simulink model "sampleModel2017"  (R2023a)
settings: Solver=VariableStepAuto  StartTime=0.0  StopTime=10.0  RelTol=1e-3
libraries: hdlsllib x4, simulink x3
settings Model: Creator=user1  LastModifiedBy=user1

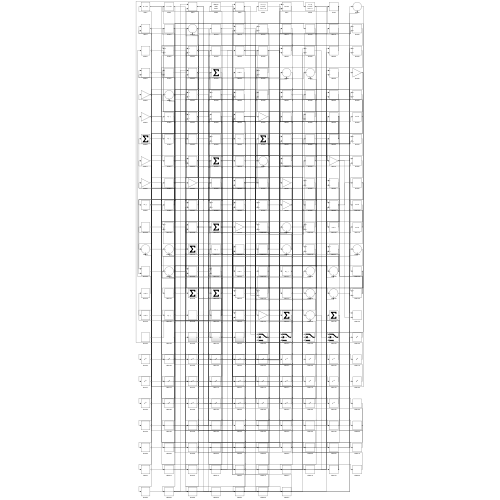
[thumbnail: Simulink's stored preview of the top-level diagram]
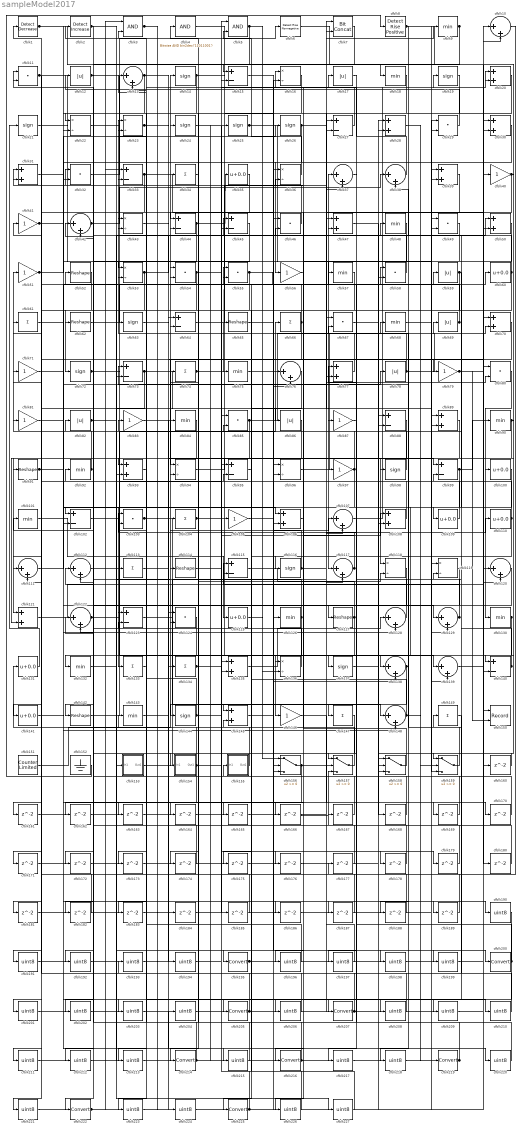
== system sampleModel2017 ==
  cfblk1 : simulink/Logic and Bit Operations/Detect Decrease  vinit=0.0  OutDataTypeStr=boolean
      settings: LibrarySourceBlock=|
      | hdlsllib/Logic and Bit
      | Operations/Detect
      | Decrease
  cfblk{10,13,37..38,42,76,107,111..112,117,120,122,128..129,138..139,148} (17 alike) : Sum  Inputs=|++
  cfblk{35,60,100,109..110,125,131,141} (8 alike) : Bias  Bias=0.0  SaturateOnIntegerOverflow=off
  cfblk{9,18,48,57,68,75,84,90,92,101,126,130,132,143} (14 alike) : MinMax
  cfblk{15,27,33,44..45,64,73,88,95,99,102,115,123,140} (14 alike) : Sum  Inputs=+-
  cfblk{11,29,32,46,49,54..55,58,67,80,85,103,124} (13 alike) : DotProduct  OutDataTypeStr=Inherit: Inherit via internal rule
  cfblk{34,61,66,74,104,113,133..134,147,149} (10 alike) : Sum  Inputs=+
  cfblk{40..41,51,56,71,79,81,83,87,97,105,146} (12 alike) : Gain
  cfblk{20,28,30..31,39,47,50,70,77,89,93,106,108,121,135,145} (16 alike) : Sum
  cfblk{52,62,65,91,114,127,142} (7 alike) : Reshape
  cfblk{14,19,21,24..26,63,72,98,116,137,144} (12 alike) : Signum
  cfblk{16,22..23,36,43,53,94,96,118..119,136} (11 alike) : Product  Inputs=*/  RndMeth=Zero  SaturateOnIntegerOverflow=on
  cfblk{12,17,59,69,78,82,86} (7 alike) : Abs  SaturateOnIntegerOverflow=off
  cfblk150 : Record  FileSettingsInternal="{\"entries\":[{\"content\":{\"excelSettings\":{\"content\":{},\"type\":\"Streamout.ExcelSettings\"}},\"type\":\"Streamout.FileSettingStorage\",\"uuid\":\"\"}],\"packageUris\":[\"http:\\/\\/schema.mathworks.com\\/mf0\\/streamout_blocks\\/R2020a\"],\"version\":\"1.0\"}"  Layout=[1 1]  SignalsInternal="{\"entries\":[{\"content\":{\"signals\":[{\"content\":{\"blockPath\":[],\"dimensions\":[1],\"domain\":\"\",\"lineColor\":\"#a2142f\",\"plots\":[1],\"port\":1,\"signalID\":5993,\"signalName\":\"XY Graph:1\"},\"type\":\"RecordBlkView.Signal\",\"uuid\":\"\"},{\"content\":{\"blockPath\":[],\"dimensions\":[1],\"domain\":\"\",\"lineColor\":\"#139fff\",\"plots\":[1],\"port\":2,\"signalID\":5996,\"signalName\":\"XY Graph:2\"},\"type\":\"RecordBlkView.Signal\",\"uuid\":\"\"}]},\"type\":\"RecordBlkView.InputSignals\",\"uuid\":\"\"}],\"packageUris\":[\"http:\\/\\/schema.mathworks.com\\/mf0\\/streamout_blocks\\/R2020a\"],\"version\":\"1.0\"}"  VisualizationBindings="{\"xyplotplugin\":{\"info\":[{\"series\":[{\"bindingParametersList\":[{\"parameter\":\"X-Axis\",\"signalID\":5993,\"signalName\":\"XY Graph:1\"},{\"parameter\":\"Y-Axis\",\"signalID\":5996,\"signalName\":\"XY Graph:2\"}],\"seriesID\":10009}],\"subplotID\":1}]}}"  CompatibilityTag=XY  st=-1
  cfblk151 : hdlsllib/Sources/Counter Limited  uplimit=7  tsamp=-1
  cfblk152 : Ground
  cfblk153 : Subsystem
      settings: LibrarySourceBlock=|
      | hdlsllib/Ports &
      | Subsystems/Subsystem
  cfblk154 : Subsystem
      settings: LibrarySourceBlock=|
      | hdlsllib/Ports &
      | Subsystems/Subsystem
  cfblk155 : Subsystem
      settings: LibrarySourceBlock=|
      | hdlsllib/Ports &
      | Subsystems/Subsystem
  cfblk{156..159} (4 alike) : Switch  SaturateOnIntegerOverflow=off  InputSameDT=off
  cfblk{160..189} (30 alike) : Delay  SampleTime=1
  cfblk{190..194,196..199,201..204,206,208..213,215,217..218,220..221,223..224,226..227} (29 alike) : DataTypeConversion  OutDataTypeStr=uint8  SaturateOnIntegerOverflow=off  RndMeth=Floor
  cfblk{195,200,205,207,214,216,219,222,225} (9 alike) : DataTypeConversion  SaturateOnIntegerOverflow=off  RndMeth=Floor
  cfblk2 : simulink/Logic and Bit Operations/Detect Increase  vinit=0.0  OutDataTypeStr=boolean
      settings: LibrarySourceBlock=|
      | hdlsllib/Logic and Bit
      | Operations/Detect
      | Increase
  cfblk3 : Logic  AllPortsSameDT=off  OutDataTypeStr=boolean
  cfblk4 : simulink/Logic and Bit Operations/Bitwise Operator  logicop=AND  UseBitMask=on  BitMask=bin2dec('11011001')  BitMaskRealWorld=Stored Integer
      settings: LibrarySourceBlock=|
      | hdlsllib/Logic and Bit
      | Operations/Bitwise
      | Operator
  cfblk5 : Logic  AllPortsSameDT=off  OutDataTypeStr=boolean
  cfblk6 : hdlsllib/Logic and Bit Operations/Detect Rise Nonnegative  vinit=0  OutDataTypeStr=boolean
  cfblk7 : hdlsllib/Logic and Bit Operations/Bit Concat  numInputs=2
  cfblk8 : hdlsllib/Logic and Bit Operations/Detect Rise Positive  vinit=0  OutDataTypeStr=boolean
  wires:
  cfblk80/1 -> cfblk130/1
  cfblk84/1 -> cfblk121/1
  cfblk26/1 -> cfblk56/1, cfblk89/2, cfblk50/2
  cfblk46/1 -> cfblk31/1
  cfblk104/1 -> cfblk129/2, cfblk178/1
  cfblk125/1 -> cfblk156/1
  cfblk143/1 -> cfblk207/1
  cfblk107/1 -> cfblk19/1
  cfblk55/1 -> cfblk37/1, cfblk73/2, cfblk98/1, cfblk138/2
  cfblk28/1 -> cfblk219/1
  cfblk50/1 -> cfblk131/1
  cfblk85/1 -> cfblk69/1, cfblk121/2, cfblk199/1
  cfblk98/1 -> cfblk14/1
  cfblk89/1 -> cfblk118/1
  cfblk8/1 -> cfblk159/1, cfblk139/2, cfblk218/1
  cfblk117/1 -> cfblk24/1, cfblk36/2
  cfblk4/1 -> cfblk146/1
  cfblk76/1 -> cfblk145/1
  cfblk134/1 -> cfblk59/1, cfblk74/1
  cfblk99/1 -> cfblk137/1, cfblk90/1
  cfblk42/1 -> cfblk38/1, cfblk210/1
  cfblk148/1 -> cfblk159/2, cfblk115/2
  cfblk92/1 -> cfblk51/1, cfblk71/1
  cfblk9/1 -> cfblk15/1, cfblk188/1
  cfblk34/1 -> cfblk214/1
  cfblk126/1 -> cfblk101/1, cfblk174/1
  cfblk74/1 -> cfblk35/1, cfblk186/1
  cfblk151/1 -> cfblk54/1
  cfblk136/1 -> cfblk92/1
  cfblk131/1 -> cfblk21/1
  cfblk72/1 -> cfblk135/2, cfblk3/1
  cfblk115/1 -> cfblk118/2
  cfblk25/1 -> cfblk117/1, cfblk77/2
  cfblk21/1 -> cfblk64/1
  cfblk140/1 -> cfblk81/1, cfblk48/1
  cfblk39/1 -> cfblk216/1
  cfblk138/1 -> cfblk68/1, cfblk144/1
  cfblk1/1 -> cfblk18/1, cfblk53/1
  cfblk54/1 -> cfblk179/1, cfblk191/1, cfblk201/1
  cfblk101/1 -> cfblk125/1
  cfblk158/1 -> cfblk16/1
  cfblk60/1 -> cfblk127/1, cfblk38/2, cfblk11/1, cfblk196/1
  cfblk122/1 -> cfblk139/1, cfblk45/1
  cfblk24/1 -> cfblk75/1
  cfblk142/1 -> cfblk66/1
  cfblk108/1 -> cfblk31/2
  cfblk70/1 -> cfblk94/1
  cfblk103/1 -> cfblk148/1, cfblk224/1
  cfblk11/1 -> cfblk89/1, cfblk141/1
  cfblk152/1 -> cfblk8/1
  cfblk63/1 -> cfblk205/1
  cfblk96/1 -> cfblk10/1
  cfblk95/1 -> cfblk225/1
  cfblk94/1 -> cfblk99/1
  cfblk5/1 -> cfblk112/2, cfblk136/2
  cfblk87/1 -> cfblk147/1
  cfblk77/1 -> cfblk54/2
  cfblk17/1 -> cfblk157/1
  cfblk12/1 -> cfblk87/1, cfblk102/1
  cfblk64/1 -> cfblk20/1
  cfblk90/1 -> cfblk140/1, cfblk171/1
  cfblk69/1 -> cfblk47/2, cfblk11/2
  cfblk100/1 -> cfblk133/1
  cfblk53/1 -> cfblk72/1, cfblk50/1
  cfblk32/1 -> cfblk6/1
  cfblk22/1 -> cfblk156/2
  cfblk20/1 -> cfblk44/1
  cfblk16/1 -> cfblk62/1
  cfblk47/1 -> cfblk158/1
  cfblk154/1(Out1) -> cfblk32/1, cfblk20/2, cfblk108/1, cfblk182/1
  cfblk121/1 -> cfblk40/1
  cfblk156/1 -> cfblk58/1, cfblk173/1
  cfblk91/1 -> cfblk106/1, cfblk53/2
  cfblk132/1 -> cfblk114/1
  cfblk19/1 -> cfblk27/2
  cfblk67/1 -> cfblk70/2
  cfblk82/1 -> cfblk86/1, cfblk198/1
  cfblk109/1 -> cfblk99/2
  cfblk83/1 -> cfblk195/1
  cfblk29/1 -> cfblk12/1
  cfblk129/1 -> cfblk77/1, cfblk115/1
  cfblk86/1 -> cfblk91/1
  cfblk153/1(Out1) -> cfblk80/2
  cfblk44/1 -> cfblk140/2, cfblk142/1
  cfblk75/1 -> cfblk30/1
  cfblk157/1 -> cfblk55/1
  cfblk35/1 -> cfblk132/1
  cfblk14/1 -> cfblk156/3, cfblk223/1
  cfblk144/1 -> cfblk23/2, cfblk104/1, cfblk3/2, cfblk176/1
  cfblk123/1 -> cfblk110/1
  cfblk18/1 -> cfblk93/1
  cfblk135/1 -> cfblk128/1
  cfblk66/1 -> cfblk23/1, cfblk106/2, cfblk181/1
  cfblk30/1 -> cfblk32/2
  cfblk73/1 -> cfblk108/2, cfblk221/1
  cfblk2/1 -> cfblk22/1, cfblk227/1
  cfblk97/1 -> cfblk61/1, cfblk102/2
  cfblk3/1 -> cfblk184/1, cfblk194/1
  cfblk65/1 -> cfblk76/1
  cfblk116/1 -> cfblk64/2, cfblk9/1, cfblk46/2
  cfblk130/1 -> cfblk162/1, cfblk163/1
  cfblk27/1 -> cfblk2/1
  cfblk155/1(Out1) -> cfblk42/1
  cfblk51/1 -> cfblk128/2, cfblk26/1
  cfblk33/1 -> cfblk126/1, cfblk111/1
  cfblk159/1 -> cfblk73/1
  cfblk79/1 -> cfblk10/2, cfblk150/2
  cfblk145/1 -> cfblk107/1
  cfblk38/1 -> cfblk17/1
  cfblk23/1 -> cfblk96/2, cfblk79/1
  cfblk93/1 -> cfblk13/2
  cfblk43/1 -> cfblk134/1
  cfblk36/1 -> cfblk5/2
  cfblk112/1 -> cfblk65/1
  cfblk13/1 -> cfblk22/2, cfblk215/1
  cfblk59/1 -> cfblk109/1, cfblk138/1, cfblk175/1
  cfblk78/1 -> cfblk43/1, cfblk30/2
  cfblk40/1 -> cfblk122/2, cfblk100/1
  cfblk45/1 -> cfblk154/1(In1)
  cfblk62/1 -> cfblk60/1
  cfblk102/1 -> cfblk123/1
  cfblk58/1 -> cfblk4/1
  cfblk71/1 -> cfblk148/2
  cfblk128/1 -> cfblk103/1
  cfblk68/1 -> cfblk159/3
  cfblk48/1 -> cfblk58/2
  cfblk127/1 -> cfblk44/2, cfblk136/1
  cfblk120/1 -> cfblk222/1
  cfblk111/1 -> cfblk78/1
  cfblk110/1 -> cfblk57/1, cfblk42/2, cfblk165/1
  cfblk113/1 -> cfblk200/1
  cfblk41/1 -> cfblk129/1, cfblk189/1
  cfblk6/1 -> cfblk150/1
  cfblk49/1 -> cfblk116/1
  cfblk160/1 -> cfblk158/2
  cfblk52/1 -> cfblk161/1
  cfblk161/1 -> cfblk47/1
  cfblk162/1 -> cfblk93/2
  cfblk163/1 -> cfblk117/2
  cfblk57/1 -> cfblk164/1
  cfblk164/1 -> cfblk27/1
  cfblk165/1 -> cfblk107/2
  cfblk106/1 -> cfblk166/1
  cfblk166/1 -> cfblk157/3
  cfblk167/1 -> cfblk112/1
  cfblk137/1 -> cfblk168/1
  cfblk168/1 -> cfblk85/2
  cfblk81/1 -> cfblk169/1
  cfblk169/1 -> cfblk5/1
  cfblk146/1 -> cfblk170/1
  cfblk170/1 -> cfblk55/2
  cfblk171/1 -> cfblk158/3
  cfblk118/1 -> cfblk172/1
  cfblk172/1 -> cfblk37/2
  cfblk173/1 -> cfblk103/2
  cfblk174/1 -> cfblk33/2
  cfblk175/1 -> cfblk16/2
  cfblk10/1 -> cfblk177/1
  cfblk177/1 -> cfblk96/1
  cfblk178/1 -> cfblk135/1
  cfblk179/1 -> cfblk145/2
  cfblk139/1 -> cfblk180/1
  cfblk180/1 -> cfblk122/1
  cfblk181/1 -> cfblk45/2
  cfblk182/1 -> cfblk111/2
  cfblk133/1 -> cfblk183/1
  cfblk183/1 -> cfblk76/2
  cfblk184/1 -> cfblk157/2
  cfblk114/1 -> cfblk185/1
  cfblk185/1 -> cfblk1/1
  cfblk186/1 -> cfblk29/2
  cfblk15/1 -> cfblk187/1
  cfblk187/1 -> cfblk13/1
  cfblk188/1 -> cfblk123/2
  cfblk189/1 -> cfblk36/1
  cfblk105/1 -> cfblk190/1
  cfblk191/1 -> cfblk105/1
  cfblk124/1 -> cfblk192/1
  cfblk192/1 -> cfblk84/1
  cfblk190/1 -> cfblk193/1
  cfblk193/1 -> cfblk124/1
  cfblk194/1 -> cfblk124/2
  cfblk195/1 -> cfblk160/1, cfblk97/1
  cfblk196/1 -> cfblk83/1
  cfblk119/1 -> cfblk197/1
  cfblk197/1 -> cfblk67/1
  cfblk198/1 -> cfblk119/1
  cfblk199/1 -> cfblk119/2
  cfblk200/1 -> cfblk67/2, cfblk213/1
  cfblk201/1 -> cfblk113/1
  cfblk7/1 -> cfblk202/1
  cfblk202/1 -> cfblk70/1
  cfblk141/1 -> cfblk203/1
  cfblk203/1 -> cfblk7/1
  cfblk204/1 -> cfblk7/2
  cfblk205/1 -> cfblk41/1, cfblk155/1(In1)
  cfblk56/1 -> cfblk206/1
  cfblk206/1 -> cfblk63/1
  cfblk207/1 -> cfblk29/1, cfblk52/1
  cfblk61/1 -> cfblk208/1
  cfblk208/1 -> cfblk143/1
  cfblk149/1 -> cfblk209/1
  cfblk209/1 -> cfblk80/1
  cfblk210/1 -> cfblk149/1
  cfblk88/1 -> cfblk211/1
  cfblk211/1 -> cfblk153/1(In1)
  cfblk147/1 -> cfblk212/1
  cfblk212/1 -> cfblk88/1
  cfblk213/1 -> cfblk88/2
  cfblk214/1 -> cfblk15/2, cfblk43/2, cfblk25/1
  cfblk215/1 -> cfblk34/1
  cfblk216/1 -> cfblk49/2, cfblk82/1
  cfblk37/1 -> cfblk217/1
  cfblk217/1 -> cfblk39/1
  cfblk218/1 -> cfblk39/2
  cfblk219/1 -> cfblk167/1, cfblk94/2
  cfblk31/1 -> cfblk220/1
  cfblk220/1 -> cfblk28/1
  cfblk221/1 -> cfblk28/2
  cfblk222/1 -> cfblk204/1, cfblk46/1, cfblk33/1
  cfblk223/1 -> cfblk120/1
  cfblk224/1 -> cfblk120/2
  cfblk225/1 -> cfblk49/1, cfblk85/1
  cfblk176/1 -> cfblk226/1
  cfblk226/1 -> cfblk95/1
  cfblk227/1 -> cfblk95/2

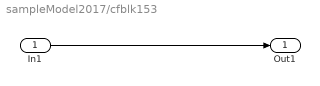
== system sampleModel2017/cfblk153 ==
  In1 : Inport
  Out1 : Outport
  wires:
  In1/1 -> Out1/1

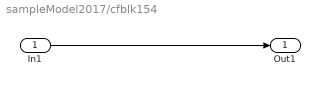
== system sampleModel2017/cfblk154 ==
  In1 : Inport
  Out1 : Outport
  wires:
  In1/1 -> Out1/1

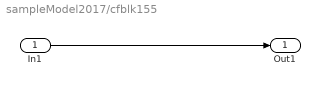
== system sampleModel2017/cfblk155 ==
  In1 : Inport
  Out1 : Outport
  wires:
  In1/1 -> Out1/1
